simulink model "INP_BRK_test"  (R2024b)
settings: Solver=VariableStepAuto  StartTime=0.0  StopTime=10.0  RelTol=1e-3
libraries: simulink x1, INP_BRK x1
settings Model: Creator=blatak  LastModifiedBy=blatak

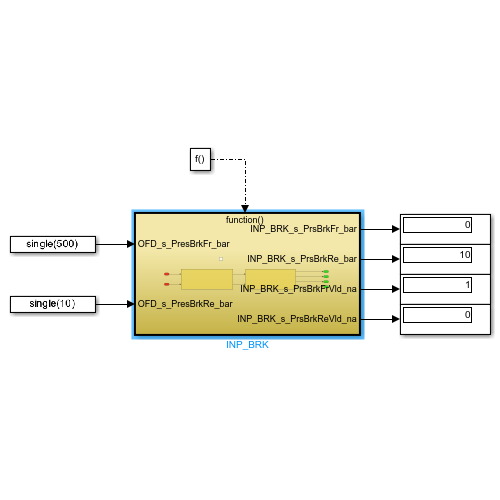
[thumbnail: Simulink's stored preview of the top-level diagram]
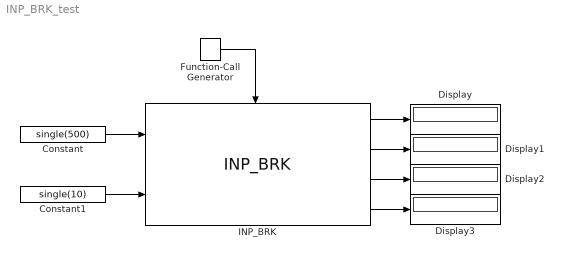
== system INP_BRK_test ==
  Constant : Constant  Value=single(500)
  Constant1 : Constant  Value=single(10)
  Display{,1..3} (4 alike) : Display
  Function-Call Generator : simulink/Ports & Subsystems/Function-Call Generator  sample_time=0.005  numberOfIterations=1  DisallowWideOutput=off
  INP_BRK : INP_BRK/INP_BRK  SystemSampleTime=-1  VariantActivationTime=update diagram  AllowFlexibleInterface=on  Latency=0  AutoFrameSizeCalculation=off
  wires:
  Constant/1 -> INP_BRK/1
  Constant1/1 -> INP_BRK/2
  INP_BRK/1 -> Display/1
  INP_BRK/2 -> Display1/1
  INP_BRK/3 -> Display2/1
  INP_BRK/4 -> Display3/1
  Function-Call Generator/1 -> INP_BRK/Trigger
